simulink model "pid_speed"  (Simulink 7.4)
settings: Solver=FixedStepDiscrete  StartTime=0.0  StopTime=100  FixedStep=0.005  RelTol=1e-3
libraries: simulink x1
settings Model: Creator=NGUYEN VINH HAO  LastModifiedBy=Admin
settings OptimizationCC: OptimizeModelRefInitCode=on  LifeSpan=1
settings HardwareCC: ProdHWDeviceType=Generic->32-bit Embedded Processor
settings RTWCC: SystemTargetFile=ert.tlc  GenCodeOnly=on  GenerateMakefile=off  TemplateMakefile=ert_default_tmf  Description=Real-Time Workshop Embedded Coder  ProcessScript=ert_make_rtw_hook
settings CodeAppCC: IgnoreCustomStorageClasses=off
settings ERTTargetCC: MultiwordLength=2048  GenerateSampleERTMain=on  ERTCustomFileTemplate=example_file_process.tlc  ConvertIfToSwitch=off

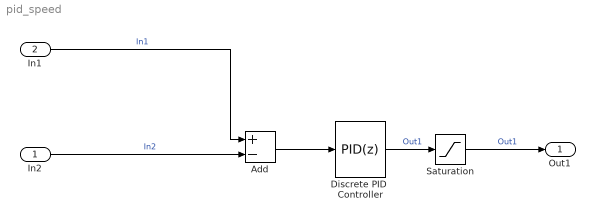
== system pid_speed ==
  In2 : Inport  OutDataType=fixdt(1, 16)  OutScaling=2^0
  In1 : Inport  Port=2  OutDataType=fixdt(1, 16)  OutScaling=2^0
  Add : Sum  Inputs=+-  OutDataType=fixdt(1, 16)  OutScaling=2^-10
  Discrete PID  Controller : simulink/Continuous/PID Controller  DialogController=pidpack.PIDConfig.pidDDGCreate  DialogControllerArgs=DataTag0  SystemSampleTime=-1  Controller=PID  TimeDomain=Discrete-time  SampleTime=-1  IntegratorMethod=Forward Euler  FilterMethod=Forward Euler  Form=Parallel  P=1  I=0.0001  D=0  N=100  InitialConditionSource=internal  InitialConditionForIntegrator=0  InitialConditionForFilter=0  ExternalReset=none  LimitOutput=off  UpperSaturationLimit=inf  LowerSaturationLimit=-inf  LinearizeAsGain=off  AntiWindupMode=none  Kb=1  TrackingMode=off  Kt=1  PParamMin=[]  PParamMax=[]  IParamMin=[]  IParamMax=[]  DParamMin=[]  DParamMax=[]  NParamMin=[]  NParamMax=[]  KbParamMin=[]  KbParamMax=[]  KtParamMin=[]  KtParamMax=[]  POutMin=[]  POutMax=[]  IOutMin=[]  IOutMax=[]  DOutMin=[]  DOutMax=[]  NOutMin=[]  NOutMax=[]  KbOutMin=[]  KbOutMax=[]  KtOutMin=[]  KtOutMax=[]  IntegratorOutMin=[]  IntegratorOutMax=[]  FilterOutMin=[]  FilterOutMax=[]  SumOutMin=[]  SumOutMax=[]  SumI1OutMin=[]  SumI1OutMax=[]  SumI2OutMin=[]  SumI2OutMax=[]  SumI3OutMin=[]  SumI3OutMax=[]  SumDOutMin=[]  SumDOutMax=[]  SaturationOutMin=[]  SaturationOutMax=[]  IntegratorContinuousStateAttributes=''  IntegratorStateMustResolveToSignalObject=off  IntegratorRTWStateStorageClass=Auto  FilterContinuousStateAttributes=''  FilterStateMustResolveToSignalObject=off  FilterRTWStateStorageClass=Auto
  Saturation : Saturate  UpperLimit=10  LowerLimit=-10  OutDataType=fixdt(1, 16)  OutScaling=2^0
  Out1 : Outport  OutDataType=fixdt(1, 16)  OutScaling=2^0
  wires:
  Discrete PID  Controller/1 -> Saturation/1  "Out1"
  Add/1 -> Discrete PID  Controller/1
  In1/1 -> Add/1  "In1"
  In2/1 -> Add/2  "In2"
  Saturation/1 -> Out1/1  "Out1"
